simulink model "Model_3_Hieu_1_12"  (R2021a)
settings: Solver=VariableStepAuto  StartTime=0.0  StopTime=10  RelTol=1e-3
InitFcn:
  | ml=0.2;
  | mc=0.5;
  | mt=0.5;
  | g=9.81;
  | l_ref=0.5;
  | l_ini=0.5;
  | l=l_ini;
  | n1=5;n2=1;
  | x_ref=10;
  | 
  | %ADRC' s parameter caculation
  | %b0 = (ml+mc)/(mc*ml +mc*mt+ml*mt); %Hieu
  | b0=(ml+mc)/(mt*mc+2*ml*mc+mt*ml+ml^2+mc^2); %Enhanced-coupling
  | k_ESO = 50;
  | T_set  = 6;
  | 
  | s_cl = -5.85/T_set;
  | Kp   = s_cl^2;
  | Kd   = -2*s_cl;
  | 
  | s_ESO = k_ESO*s_cl;
  | l1        = -3*s_ESO;
  | l2        = 3*( s_ESO)^2;
  | l3        = -(s_ESO)^3;
  | 
  | %Observer
  | A = [-l1, 1, 0;
  |         -l2, 0, 1;
  |         -l3, 0, 0];
  | B = [0;
  |         b0;
  |         0];
  | L = [l1;
  |        l2;
  |        l3];
  | 
  | %b1 = (mt+mc)/(mc*ml +mc*mt+ml*mt);
  | b1=1/(ml+mc);
  | k_ESO1 =100;
  | T_set1  = 3;
  | s_cl1 = -5.85/T_set1;
  | Kp1   = s_cl1^2;
  | Kd1   = -2*s_cl1;
  | 
  | s_ESO1 = k_ESO1*s_cl1;
  | l11        = -3*s_ESO1;
  | l21        = 3*( s_ESO1)^2;
  | l31        = -(s_ESO1)^3;
  | 
  | %Observer
  | A1 = [-l11, 1, 0;
  |         -l21, 0, 1;
  |         -l31, 0, 0];
  | B1 = [0;
  |         b1;
  |         0];
  | L1 = [l11;
  |        l21;
  |        l31];
  | 
  | ... (+35 lines)
values from neighbouring files (symbols this model uses):
  particle = repmat(empty_particle, nPop, 1)    [PSO16_12.m]    (also in PSO_ZVD.m)
undefined symbols (not defined in the file or in its folder): i
libraries: neural x35, simulink_extras x11, simulink x5
(part 12 of 15)

== matlab function Model_3_Hieu_1_12/test_RBF_1 PSO/con lắc đôi2/Crane ==
  data: dx1 output; d1x input; l1 input; d1l1 input; the1 input; d1the1 input; the2 input; d1the2 input; Fx input; Fl input; dx2 output; dx3 output; dx4 output; dx5 output; dx6 output; m2 input; dx7 output; dx8 output
function [dx1,dx2,dx3,dx4,dx5,dx6,dx7,dx8] = fcn(d1x,l1,d1l1,the1,d1the1,the2,d1the2,Fx,Fl,m2)
 m =5; m1 =2; g =9.81; l2=0.5;

 dx1=d1x;

 dx2 = (Fx*m2*cos(the1 - the2)^2 - Fx*m2 - Fx*m1 + Fx*m2*sin(the1 - the2)^2 + Fl*m1*sin(the1) + Fl*m2*sin(the1) - Fl*m2*sin(the1 - the2)*cos(the2) - d1the2^2*l2*m2^2*sin(the2) - g*m2^2*cos(the2)*sin(the2) - Fl*m2*cos(the1 - the2)^2*sin(the1) - g*m2^2*cos(the1 - the2)*sin(the1 - the2)*sin(the1)^2 + Fl*m2*cos(the1 - the2)*sin(the1 - the2)*cos(the1) + d1the2^2*l2*m2^2*cos(the1 - the2)*sin(the1) - d1the2^2*l2*m2^2*sin(the1 - the2)*cos(the1) - d1the2^2*l2*m1*m2*sin(the2) + g*m2^2*cos(the1 - the2)*cos(the1)*sin(the2) + g*m2^2*cos(the1 - the2)*cos(the2)*sin(the1) - g*m2^2*sin(the1 - the2)*cos(the1)*cos(the2) - g*m1*m2*cos(the2)*sin(the2) + g*m2^2*sin(the1 - the2)*sin(the1)*sin(the2) + d1the2^2*l2*m2^2*cos(the1 - the2)^2*sin(the2) - d1the2^2*l2*m2^2*cos(the1 - the2)^3*sin(the1) + d1the2^2*l2*m2^2*sin(the1 - the2)^3*cos(the1) - g*m2^2*cos(the1 - the2)^2*cos(the1)*sin(the1) + d1the2^2*l2*m2^2*sin(the1 - the2)^2*sin(the2) + g*m2^2*sin(the1 - the2)^2*cos(the1)*sin(the1) + g*m2^2*cos(the1 - the2)*sin(the1 - the2)*cos(the1)^2 - g*m1*m2*cos(the1 - the2)*sin(the1 - the2)*sin(the1)^2 + d1the2^2*l2*m1*m2*cos(the1 - the2)*sin(the1) - d1the2^2*l2*m1*m2*sin(the1 - the2)*cos(the1) + g*m1*m2*cos(the1 - the2)*cos(the1)*sin(the2) + g*m1*m2*cos(the1 - the2)*cos(the2)*sin(the1) - g*m1*m2*sin(the1 - the2)*cos(the1)*cos(the2) + g*m1*m2*sin(the1 - the2)*sin(the1)*sin(the2) + d1the2^2*l2*m2^2*cos(the1 - the2)^2*sin(the1 - the2)*cos(the1) - d1the2^2*l2*m2^2*cos(the1 - the2)*sin(the1 - the2)^2*sin(the1) - g*m1*m2*cos(the1 - the2)^2*cos(the1)*sin(the1) + g*m1*m2*sin(the1 - the2)^2*cos(the1)*sin(the1) + g*m1*m2*cos(the1 - the2)*sin(the1 - the2)*cos(the1)^2)/(m1^2*cos(the1)^2 - m*m2 - 2*m1*m2 - m*m1 + m2^2*cos(the1)^2 + m2^2*cos(the2)^2 + m1^2*sin(the1)^2 + m2^2*sin(the1)^2 + m2^2*cos(the1 - the2)^2 + m2^2*sin(the1 - the2)^2 - m1^2 - m2^2 + 2*m1*m2*cos(the1)^2 + m1*m2*cos(the2)^2 + 2*m1*m2*sin(the1)^2 + m*m2*cos(the1 - the2)^2 + m1*m2*cos(the1 - the2)^2 + m*m2*sin(the1 - the2)^2 + m1*m2*sin(the1 - the2)^2 - m2^2*cos(the1 - the2)^2*sin(the1)^2 - m2^2*sin(the1 - the2)^2*cos(the1)^2 - 2*m2^2*sin(the1 - the2)*cos(the2)*sin(the1) - 2*m2^2*cos(the1 - the2)*cos(the1)*cos(the2) - m1*m2*cos(the1 - the2)^2*sin(the1)^2 - m1*m2*sin(the1 - the2)^2*cos(the1)^2 + 2*m2^2*cos(the1 - the2)*sin(the1 - the2)*cos(the1)*sin(the1) - 2*m1*m2*sin(the1 - the2)*cos(the2)*sin(the1) - 2*m1*m2*cos(the1 - the2)*cos(the1)*cos(the2) + 2*m1*m2*cos(the1 - the2)*sin(the1 - the2)*cos(the1)*sin(the1));

 %d2x = -(Fx*m1 + Fx*m2 + g*m1^2*sin(the1) + g*m2^2*sin(the1) - Fx*m2*cos(the1 - the2)^2 - Fx*m2*sin(the1 - the2)^2 - Fl*m1*sin(the1) - Fl*m2*sin(the1) + Fl*m2*sin(the1 - the2)*cos(the2) + d1the2^2*l2*m2^2*sin(the2) - g*m1^2*cos(the1)*sin(the1) - g*m2^2*cos(the1)*sin(the1) + g*m2^2*cos(the2)*sin(the2) + Fl*m2*cos(the1 - the2)^2*sin(the1) - g*m2^2*sin(the1 - the2)*cos(the2) + 2*g*m1*m2*sin(the1) - g*m2^2*cos(the1 - the2)^2*sin(the1) - Fl*m2*cos(the1 - the2)*sin(the1 - the2)*cos(the1) + 2*d1l1*d1the1*m2^2*cos(the1 - the2)^2*cos(the1) - 2*d1l1*d1the1*m2^3*cos(the1 - the2)^2*cos(the1) + d1the2^2*l2*m2^2*cos(the1 - the2)*sin(the1) + d1the2^2*l2*m2^2*sin(the1 - the2)*cos(the1) + d1the2^2*l2*m1*m2*sin(the2) - g*m2^2*cos(the1 - the2)*cos(the1)*sin(the2) + g*m2^2*sin(the1 - the2)*cos(the1)*cos(the2) - 2*g*m1*m2*cos(the1)*sin(the1) + g*m1*m2*cos(the2)*sin(the2) - g*m2^2*sin(the1 - the2)*sin(the1)*sin(the2) + g*m2^2*cos(the1 - the2)*sin(the1 - the2)*cos(the1) - g*m1*m2*sin(the1 - the2)*cos(the2) - d1the2^2*l2*m2^2*cos(the1 - the2)^2*sin(the2) - d1the2^2*l2*m2^2*cos(the1 - the2)^3*sin(the1) - d1the2^2*l2*m2^2*sin(the1 - the2)^3*cos(the1) + g*m2^2*cos(the1 - the2)^2*cos(the1)*sin(the1) - d1the2^2*l2*m2^2*sin(the1 - the2)^2*sin(the2) - 2*d1l1*d1the1*m2^2*cos(the1 - the2)*cos(the2) + 2*d1l1*d1the1*m2^3*cos(the1 - the2)*cos(the2) - g*m2^2*cos(the1 - the2)*sin(the1 - the2)*cos(the1)^2 - g*m1*m2*cos(the1 - the2)^2*sin(the1) + 2*d1l1*d1the1*m2^2*cos(the1 - the2)*sin(the1 - the2)*sin(the1) - 2*d1l1*d1the1*m2^3*cos(the1 - the2)*sin(the1 - the2)*sin(the1) + 2*d1l1*d1the1*m1*m2*cos(the1 - the2)^2*cos(the1) + 2*d1l1*d1the1*m1*m2^2*cos(the1 - the2)*cos(the2) - 2*d1the2^2*l2*m2^2*cos(the1 - the2)*sin(the1 - the2)*cos(the2) + d1the2^2*l2*m1*m2*cos(the1 - the2)*sin(the1) + d1the2^2*l2*m1*m2*sin(the1 - the2)*cos(the1) - g*m1*m2*cos(the1 - the2)*cos(the1)*sin(the2) + g*m1*m2*sin(the1 - the2)*cos(the1)*cos(the2) - g*m1*m2*sin(the1 - the2)*sin(the1)*sin(the2) + g*m1*m2*cos(the1 - the2)*sin(the1 - the2)*cos(the1) - 2*d1l1*d1the1*m1*m2^2*cos(the1 - the2)^2*cos(the1) + d1the2^2*l2*m2^2*cos(the1 - the2)^2*sin(the1 - the2)*cos(the1) + d1the2^2*l2*m2^2*cos(the1 - the2)*sin(the1 - the2)^2*sin(the1) + g*m1*m2*cos(the1 - the2)^2*cos(the1)*sin(the1) - 2*d1l1*d1the1*m1*m2*cos(the1 - the2)*cos(the2) - g*m1*m2*cos(the1 - the2)*sin(the1 - the2)*cos(the1)^2 + 2*d1l1*d1the1*m1*m2*cos(the1 - the2)*sin(the1 - the2)*sin(the1) - 2*d1l1*d1the1*m1*m2^2*cos(the1 - the2)*sin(the1 - the2)*sin(the1))/(m1^2*cos(the1)^2 - m*m2 - 2*m1*m2 - m*m1 + m2^2*cos(the1)^2 + m2^2*cos(the2)^2 + m1^2*sin(the1)^2 + m2^2*sin(the1)^2 + m2^2*cos(the1 - the2)^2 + m2^2*sin(the1 - the2)^2 - m1^2 - m2^2 + 2*m1*m2*cos(the1)^2 + m1*m2*cos(the2)^2 + 2*m1*m2*sin(the1)^2 + m*m2*cos(the1 - the2)^2 + m1*m2*cos(the1 - the2)^2 + m*m2*sin(the1 - the2)^2 + m1*m2*sin(the1 - the2)^2 - m2^2*cos(the1 - the2)^2*sin(the1)^2 - m2^2*sin(the1 - the2)^2*cos(the1)^2 - 2*m2^2*sin(the1 - the2)*cos(the2)*sin(the1) - 2*m2^2*cos(the1 - the2)*cos(the1)*cos(the2) - m1*m2*cos(the1 - the2)^2*sin(the1)^2 - m1*m2*sin(the1 - the2)^2*cos(the1)^2 + 2*m2^2*cos(the1 - the2)*sin(the1 - the2)*cos(the1)*sin(the1) - 2*m1*m2*sin(the1 - the2)*cos(the2)*sin(the1) - 2*m1*m2*cos(the1 - the2)*cos(the1)*cos(the2) + 2*m1*m2*cos(the1 - the2)*sin(the1 - the2)*cos(the1)*sin(the1));

 dx3=d1l1;

 dx4 = (Fx*m1^2*sin(the1) - Fl*m2^2 - Fl*m1^2 + Fx*m2^2*sin(the1) - d1the1^2*l1*m1^3 - d1the1^2*l1*m2^3 - g*m1^3*cos(the1) - g*m2^3*cos(the1) - Fl*m*m1 - Fl*m*m2 - 2*Fl*m1*m2 + Fl*m1^2*cos(the1)^2 + Fl*m2^2*cos(the1)^2 + Fl*m2^2*cos(the2)^2 + g*m1^3*cos(the1)^3 + g*m2^3*cos(the1)^3 + Fl*m2^2*cos(the1 - the2)^2 + 3*g*m1*m2^2*cos(the1)^3 + 3*g*m1^2*m2*cos(the1)^3 - Fx*m2^2*sin(the1 - the2)*cos(the2) - d1the2^2*l2*m2^3*cos(the1 - the2) + 2*Fx*m1*m2*sin(the1) + d1the1^2*l1*m1^3*cos(the1)^2 + d1the1^2*l1*m2^3*cos(the1)^2 + d1the1^2*l1*m2^3*cos(the2)^2 - g*m2^3*sin(the1 - the2)*sin(the2) + g*m2^3*cos(the1)*cos(the2)^2 + d1the1^2*l1*m1^3*sin(the1)^2 + d1the1^2*l1*m2^3*sin(the1)^2 + g*m1^3*cos(the1)*sin(the1)^2 + g*m2^3*cos(the1)*sin(the1)^2 + 2*Fl*m1*m2*cos(the1)^2 + Fl*m1*m2*cos(the2)^2 - Fx*m2^2*cos(the1 - the2)^2*sin(the1) + d1the1^2*l1*m2^3*cos(the1 - the2)^2 + d1the2^2*l2*m2^3*cos(the1 - the2)^3 - d1the1^2*l1*m*m1^2 - d1the1^2*l1*m*m2^2 - 3*d1the1^2*l1*m1*m2^2 - 3*d1the1^2*l1*m1^2*m2 + g*m2^3*cos(the1 - the2)^2*cos(the1) + d1the1^2*l1*m2^3*sin(the1 - the2)^2 - g*m*m1^2*cos(the1) - g*m*m2^2*cos(the1) - 3*g*m1*m2^2*cos(the1) - 3*g*m1^2*m2*cos(the1) + Fl*m*m2*cos(the1 - the2)^2 + Fl*m1*m2*cos(the1 - the2)^2 - g*m*m2^2*sin(the1 - the2)*sin(the2) - 2*g*m1*m2^2*sin(the1 - the2)*sin(the2) - g*m1^2*m2*sin(the1 - the2)*sin(the2) - d1the1^2*l1*m2^3*cos(the1 - the2)^2*sin(the1)^2 - d1the1^2*l1*m2^3*sin(the1 - the2)^2*cos(the1)^2 + 2*g*m1*m2^2*cos(the1)*cos(the2)^2 + g*m1^2*m2*cos(the1)*cos(the2)^2 + 3*d1the1^2*l1*m1*m2^2*sin(the1)^2 + 3*d1the1^2*l1*m1^2*m2*sin(the1)^2 + 3*g*m1*m2^2*cos(the1)*sin(the1)^2 + 3*g*m1^2*m2*cos(the1)*sin(the1)^2 + d1the2^2*l2*m2^3*sin(the1)*sin(the2) - 2*Fl*m2^2*cos(the1 - the2)*cos(the1)*cos(the2) + d1the1^2*l1*m*m2^2*cos(the1 - the2)^2 + 2*d1the1^2*l1*m1*m2^2*cos(the1 - the2)^2 + d1the1^2*l1*m1^2*m2*cos(the1 - the2)^2 + d1the2^2*l2*m*m2^2*cos(the1 - the2)^3 + d1the2^2*l2*m1*m2^2*cos(the1 - the2)^3 + g*m2^3*cos(the2)*sin(the1)*sin(the2) + g*m*m2^2*cos(the1 - the2)^2*cos(the1) + 2*g*m1*m2^2*cos(the1 - the2)^2*cos(the1) + g*m1^2*m2*cos(the1 - the2)^2*cos(the1) + d1the1^2*l1*m*m2^2*sin(the1 - the2)^2 + 2*d1the1^2*l1*m1*m2^2*sin(the1 - the2)^2 + d1the1^2*l1*m1^2*m2*sin(the1 - the2)^2 + Fx*m2^2*cos(the1 - the2)*sin(the1 - the2)*cos(the1) - Fx*m1*m2*sin(the1 - the2)*cos(the2) + d1the2^2*l2*m2^3*cos(the1 - the2)*cos(the1)^2 + d1the2^2*l2*m2^3*cos(the1 - the2)*cos(the2)^2 + g*m2^3*cos(the1 - the2)*sin(the1 - the2)*sin(the1) - 2*g*m2^3*cos(the1 - the2)*cos(the1)^2*cos(the2) - g*m2^3*cos(the1 - the2)*cos(the2)*sin(the1)^2 + g*m2^3*sin(the1 - the2)*cos(the1)^2*sin(the2) - Fx*m1*m2*cos(the1 - the2)^2*sin(the1) - d1the2^2*l2*m*m2^2*cos(the1 - the2) - 2*d1the2^2*l2*m1*m2^2*cos(the1 - the2) - d1the2^2*l2*m1^2*m2*cos(the1 - the2) - 2*d1the1^2*l1*m*m1*m2 + d1the2^2*l2*m2^3*cos(the1 - the2)*sin(the1 - the2)^2 - 2*g*m*m1*m2*cos(the1) + 3*d1the1^2*l1*m1*m2^2*cos(the1)^2 + 3*d1the1^2*l1*m1^2*m2*cos(the1)^2 + 2*d1the1^2*l1*m1*m2^2*cos(the2)^2 + d1the1^2*l1*m1^2*m2*cos(the2)^2 + 2*d1the2^2*l2*m1*m2^2*cos(the1 - the2)*cos(the1)^2 + d1the2^2*l2*m1^2*m2*cos(the1 - the2)*cos(the1)^2 + d1the2^2*l2*m1*m2^2*cos(the1 - the2)*cos(the2)^2 + g*m*m2^2*cos(the1 - the2)*sin(the1 - the2)*sin(the1) + 2*g*m1*m2^2*cos(the1 - the2)*sin(the1 - the2)*sin(the1) + g*m1^2*m2*cos(the1 - the2)*sin(the1 - the2)*sin(the1) - g*m*m1*m2*sin(the1 - the2)*sin(the2) - 2*d1the1^2*l1*m2^3*cos(the1 - the2)*cos(the1)*cos(the2) - 4*g*m1*m2^2*cos(the1 - the2)*cos(the1)^2*cos(the2) - 2*g*m1^2*m2*cos(the1 - the2)*cos(the1)^2*cos(the2) - 2*g*m1*m2^2*cos(the1 - the2)*cos(the2)*sin(the1)^2 - g*m1^2*m2*cos(the1 - the2)*cos(the2)*sin(the1)^2 - 2*d1the1^2*l1*m2^3*sin(the1 - the2)*cos(the2)*sin(the1) + d1the2^2*l2*m2^3*sin(the1 - the2)*cos(the1)*sin(the1) - d1the2^2*l2*m2^3*sin(the1 - the2)*cos(the2)*sin(the2) + 2*g*m1*m2^2*sin(the1 - the2)*cos(the1)^2*sin(the2) + g*m1^2*m2*sin(the1 - the2)*cos(the1)^2*sin(the2) - 2*Fl*m1*m2*cos(the1 - the2)*cos(the1)*cos(the2) + d1the1^2*l1*m*m1*m2*cos(the1 - the2)^2 - g*m2^3*cos(the1 - the2)*cos(the1)*sin(the1)*sin(the2) - g*m2^3*sin(the1 - the2)*cos(the1)*cos(the2)*sin(the1) + d1the2^2*l2*m*m2^2*cos(the1 - the2)*sin(the1 - the2)^2 + d1the2^2*l2*m1*m2^2*cos(the1 - the2)*sin(the1 - the2)^2 + g*m*m1*m2*cos(the1 - the2)^2*cos(the1) + d1the1^2*l1*m*m1*m2*sin(the1 - the2)^2 - 2*d1the2^2*l2*m2^3*cos(the1 - the2)^2*cos(the1)*cos(the2) - 2*d1the1^2*l1*m1*m2^2*cos(the1 - the2)^2*sin(the1)^2 - 2*d1the1^2*l1*m1*m2^2*sin(the1 - the2)^2*cos(the1)^2 - d1the1^2*l1*m1^2*m2*cos(the1 - the2)^2*sin(the1)^2 - d1the1^2*l1*m1^2*m2*sin(the1 - the2)^2*cos(the1)^2 + Fx*m1*m2*cos(the1 - the2)*sin(the1 - the2)*cos(the1) - d1the2^2*l2*m2^3*sin(the1 - the2)^2*cos(the1)*cos(the2) - d1the2^2*l2*m2^3*cos(the1 - the2)^2*sin(the1)*sin(the2) + 2*d1the2^2*l2*m1*m2^2*sin(the1)*sin(the2) + d1the2^2*l2*m1^2*m2*sin(the1)*sin(the2) + 2*g*m1*m2^2*cos(the2)*sin(the1)*sin(the2) + g*m1^2*m2*cos(the2)*sin(the1)*sin(the2) - d1the2^2*l2*m*m1*m2*cos(the1 - the2) - d1the2^2*l2*m1*m2^2*cos(the1 - the2)^2*sin(the1)*sin(the2) + g*m*m1*m2*cos(the1 - the2)*sin(the1 - the2)*sin(the1) + 2*d1the1^2*l1*m2^3*cos(the1 - the2)*sin(the1 - the2)*cos(the1)*sin(the1) + d1the2^2*l2*m2^3*cos(the1 - the2)*sin(the1 - the2)*cos(the1)*sin(the2) - d1the2^2*l2*m2^3*cos(the1 - the2)*sin(the1 - the2)*cos(the2)*sin(the1) - 4*d1the1^2*l1*m1*m2^2*cos(the1 - the2)*cos(the1)*cos(the2) - 2*d1the1^2*l1*m1^2*m2*cos(the1 - the2)*cos(the1)*cos(the2) - 4*d1the1^2*l1*m1*m2^2*sin(the1 - the2)*cos(the2)*sin(the1) - 2*d1the1^2*l1*m1^2*m2*sin(the1 - the2)*cos(the2)*sin(the1) + 2*d1the2^2*l2*m1*m2^2*sin(the1 - the2)*cos(the1)*sin(the1) + d1the2^2*l2*m1^2*m2*sin(the1 - the2)*cos(the1)*sin(the1) - d1the2^2*l2*m1*m2^2*sin(the1 - the2)*cos(the2)*sin(the2) - 2*g*m1*m2^2*cos(the1 - the2)*cos(the1)*sin(the1)*sin(the2) - 2*g*m1*m2^2*sin(the1 - the2)*cos(the1)*cos(the2)*sin(the1) - g*m1^2*m2*cos(the1 - the2)*cos(the1)*sin(the1)*sin(the2) - g*m1^2*m2*sin(the1 - the2)*cos(the1)*cos(the2)*sin(the1) - 2*d1the2^2*l2*m1*m2^2*cos(the1 - the2)^2*cos(the1)*cos(the2) - d1the2^2*l2*m1*m2^2*sin(the1 - the2)^2*cos(the1)*cos(the2) + 4*d1the1^2*l1*m1*m2^2*cos(the1 - the2)*sin(the1 - the2)*cos(the1)*sin(the1) + 2*d1the1^2*l1*m1^2*m2*cos(the1 - the2)*sin(the1 - the2)*cos(the1)*sin(the1) + d1the2^2*l2*m1*m2^2*cos(the1 - the2)*sin(the1 - the2)*cos(the1)*sin(the2) - d1the2^2*l2*m1*m2^2*cos(the1 - the2)*sin(the1 - the2)*cos(the2)*sin(the1))/((m1 + m2)*(m1^2*cos(the1)^2 - m*m2 - 2*m1*m2 - m*m1 + m2^2*cos(the1)^2 + m2^2*cos(the2)^2 + m1^2*sin(the1)^2 + m2^2*sin(the1)^2 + m2^2*cos(the1 - the2)^2 + m2^2*sin(the1 - the2)^2 - m1^2 - m2^2 + 2*m1*m2*cos(the1)^2 + m1*m2*cos(the2)^2 + 2*m1*m2*sin(the1)^2 + m*m2*cos(the1 - the2)^2 + m1*m2*cos(the1 - the2)^2 + m*m2*sin(the1 - the2)^2 + m1*m2*sin(the1 - the2)^2 - m2^2*cos(the1 - the2)^2*sin(the1)^2 - m2^2*sin(the1 - the2)^2*cos(the1)^2 - 2*m2^2*sin(the1 - the2)*cos(the2)*sin(the1) - 2*m2^2*cos(the1 - the2)*cos(the1)*cos(the2) - m1*m2*cos(the1 - the2)^2*sin(the1)^2 - m1*m2*sin(the1 - the2)^2*cos(the1)^2 + 2*m2^2*cos(the1 - the2)*sin(the1 - the2)*cos(the1)*sin(the1) - 2*m1*m2*sin(the1 - the2)*cos(the2)*sin(the1) - 2*m1*m2*cos(the1 - the2)*cos(the1)*cos(the2) + 2*m1*m2*cos(the1 - the2)*sin(the1 - the2)*cos(the1)*sin(the1)));

 %dx4 = (g*m1^3 - Fl*m2^2 - Fl*m1^2 + g*m2^3 + Fx*m1^2*sin(the1) + Fx*m2^2*sin(the1) - d1the1^2*l1*m1^3 - d1the1^2*l1*m2^3 - g*m1^3*cos(the1) - g*m2^3*cos(the1) - Fl*m*m1 - Fl*m*m2 - 2*Fl*m1*m2 + Fl*m1^2*cos(the1)^2 + Fl*m2^2*cos(the1)^2 + Fl*m2^2*cos(the2)^2 - g*m1^3*cos(the1)^2 + g*m1^3*cos(the1)^3 - g*m2^3*cos(the1)^2 + g*m2^3*cos(the1)^3 - g*m2^3*cos(the2)^2 + Fl*m2^2*cos(the1 - the2)^2 - g*m2^3*cos(the1 - the2)^2 + g*m*m1^2 + g*m*m2^2 + 3*g*m1*m2^2 + 3*g*m1^2*m2 + 2*g*m*m1*m2 - 3*g*m1*m2^2*cos(the1)^2 - 3*g*m1^2*m2*cos(the1)^2 + 3*g*m1*m2^2*cos(the1)^3 - 2*g*m1*m2^2*cos(the2)^2 + 3*g*m1^2*m2*cos(the1)^3 - g*m1^2*m2*cos(the2)^2 - Fx*m2^2*sin(the1 - the2)*cos(the2) + d1the2^2*l2*m2^3*cos(the1 - the2) + 2*Fx*m1*m2*sin(the1) - g*m*m2^2*cos(the1 - the2)^2 - 2*g*m1*m2^2*cos(the1 - the2)^2 - g*m1^2*m2*cos(the1 - the2)^2 + d1the1^2*l1*m1^3*cos(the1)^2 + d1the1^2*l1*m2^3*cos(the1)^2 + d1the1^2*l1*m2^3*cos(the2)^2 - g*m2^3*sin(the1 - the2)*sin(the2) + g*m2^3*cos(the1)*cos(the2)^2 + d1the1^2*l1*m1^3*sin(the1)^2 + d1the1^2*l1*m2^3*sin(the1)^2 + 2*Fl*m1*m2*cos(the1)^2 + Fl*m1*m2*cos(the2)^2 - Fx*m2^2*cos(the1 - the2)^2*sin(the1) + d1the1^2*l1*m2^3*cos(the1 - the2)^2 - d1the2^2*l2*m2^3*cos(the1 - the2)^3 - d1the1^2*l1*m*m1^2 - d1the1^2*l1*m*m2^2 - 3*d1the1^2*l1*m1*m2^2 - 3*d1the1^2*l1*m1^2*m2 + g*m2^3*cos(the1 - the2)^2*cos(the1) + d1the1^2*l1*m2^3*sin(the1 - the2)^2 - g*m*m1^2*cos(the1) - g*m*m2^2*cos(the1) - 3*g*m1*m2^2*cos(the1) - 3*g*m1^2*m2*cos(the1) + Fl*m*m2*cos(the1 - the2)^2 + Fl*m1*m2*cos(the1 - the2)^2 - g*m*m2^2*sin(the1 - the2)*sin(the2) - 2*g*m1*m2^2*sin(the1 - the2)*sin(the2) - g*m1^2*m2*sin(the1 - the2)*sin(the2) - d1the1^2*l1*m2^3*cos(the1 - the2)^2*sin(the1)^2 - d1the1^2*l1*m2^3*sin(the1 - the2)^2*cos(the1)^2 + 2*g*m1*m2^2*cos(the1)*cos(the2)^2 + g*m1^2*m2*cos(the1)*cos(the2)^2 + 3*d1the1^2*l1*m1*m2^2*sin(the1)^2 + 3*d1the1^2*l1*m1^2*m2*sin(the1)^2 + 2*d1l1*d1the1*m2^3*cos(the1 - the2)*sin(the1 - the2) - 2*d1l1*d1the1*m2^4*cos(the1 - the2)*sin(the1 - the2) + d1the2^2*l2*m2^3*sin(the1)*sin(the2) - 2*Fl*m2^2*cos(the1 - the2)*cos(the1)*cos(the2) + d1the1^2*l1*m*m2^2*cos(the1 - the2)^2 + 2*d1the1^2*l1*m1*m2^2*cos(the1 - the2)^2 + d1the1^2*l1*m1^2*m2*cos(the1 - the2)^2 - d1the2^2*l2*m*m2^2*cos(the1 - the2)^3 - d1the2^2*l2*m1*m2^2*cos(the1 - the2)^3 + g*m2^3*cos(the2)*sin(the1)*sin(the2) + g*m*m2^2*cos(the1 - the2)^2*cos(the1) + 2*g*m1*m2^2*cos(the1 - the2)^2*cos(the1) + g*m1^2*m2*cos(the1 - the2)^2*cos(the1) + d1the1^2*l1*m*m2^2*sin(the1 - the2)^2 + 2*d1the1^2*l1*m1*m2^2*sin(the1 - the2)^2 + d1the1^2*l1*m1^2*m2*sin(the1 - the2)^2 + 2*g*m2^3*cos(the1 - the2)*cos(the1)*cos(the2) + Fx*m2^2*cos(the1 - the2)*sin(the1 - the2)*cos(the1) - Fx*m1*m2*sin(the1 - the2)*cos(the2) - g*m*m1*m2*cos(the1 - the2)^2 - d1the2^2*l2*m2^3*cos(the1 - the2)*cos(the1)^2 - d1the2^2*l2*m2^3*cos(the1 - the2)*cos(the2)^2 - 2*g*m2^3*cos(the1 - the2)*cos(the1)^2*cos(the2) + g*m2^3*sin(the1 - the2)*cos(the1)^2*sin(the2) - Fx*m1*m2*cos(the1 - the2)^2*sin(the1) + d1the2^2*l2*m*m2^2*cos(the1 - the2) + 2*d1the2^2*l2*m1*m2^2*cos(the1 - the2) + d1the2^2*l2*m1^2*m2*cos(the1 - the2) - 2*d1the1^2*l1*m*m1*m2 + d1the2^2*l2*m2^3*cos(the1 - the2)*sin(the1 - the2)^2 - 2*g*m*m1*m2*cos(the1) + 3*d1the1^2*l1*m1*m2^2*cos(the1)^2 + 3*d1the1^2*l1*m1^2*m2*cos(the1)^2 + 2*d1the1^2*l1*m1*m2^2*cos(the2)^2 + d1the1^2*l1*m1^2*m2*cos(the2)^2 - 2*d1the2^2*l2*m1*m2^2*cos(the1 - the2)*cos(the1)^2 - d1the2^2*l2*m1^2*m2*cos(the1 - the2)*cos(the1)^2 - d1the2^2*l2*m1*m2^2*cos(the1 - the2)*cos(the2)^2 - g*m*m1*m2*sin(the1 - the2)*sin(the2) - 2*d1the1^2*l1*m2^3*cos(the1 - the2)*cos(the1)*cos(the2) - 4*g*m1*m2^2*cos(the1 - the2)*cos(the1)^2*cos(the2) - 2*g*m1^2*m2*cos(the1 - the2)*cos(the1)^2*cos(the2) + 2*d1l1*d1the1*m2^3*cos(the1 - the2)^2*cos(the1)*sin(the1) - 2*d1l1*d1the1*m2^4*cos(the1 - the2)^2*cos(the1)*sin(the1) - 2*d1the1^2*l1*m2^3*sin(the1 - the2)*cos(the2)*sin(the1) + d1the2^2*l2*m2^3*sin(the1 - the2)*cos(the1)*sin(the1) - d1the2^2*l2*m2^3*sin(the1 - the2)*cos(the2)*sin(the2) + 2*g*m1*m2^2*sin(the1 - the2)*cos(the1)^2*sin(the2) + g*m1^2*m2*sin(the1 - the2)*cos(the1)^2*sin(the2) - 2*Fl*m1*m2*cos(the1 - the2)*cos(the1)*cos(the2) + d1the1^2*l1*m*m1*m2*cos(the1 - the2)^2 - g*m2^3*cos(the1 - the2)*cos(the1)*sin(the1)*sin(the2) + d1the2^2*l2*m*m2^2*cos(the1 - the2)*sin(the1 - the2)^2 + d1the2^2*l2*m1*m2^2*cos(the1 - the2)*sin(the1 - the2)^2 + g*m*m1*m2*cos(the1 - the2)^2*cos(the1) + d1the1^2*l1*m*m1*m2*sin(the1 - the2)^2 - 2*d1l1*d1the1*m2^3*cos(the1 - the2)*sin(the1 - the2)*cos(the1)^2 + 2*d1l1*d1the1*m2^4*cos(the1 - the2)*sin(the1 - the2)*cos(the1)^2 + 2*d1the2^2*l2*m2^3*cos(the1 - the2)^2*cos(the1)*cos(the2) - 2*d1the1^2*l1*m1*m2^2*cos(the1 - the2)^2*sin(the1)^2 - 2*d1the1^2*l1*m1*m2^2*sin(the1 - the2)^2*cos(the1)^2 - d1the1^2*l1*m1^2*m2*cos(the1 - the2)^2*sin(the1)^2 - d1the1^2*l1*m1^2*m2*sin(the1 - the2)^2*cos(the1)^2 + Fx*m1*m2*cos(the1 - the2)*sin(the1 - the2)*cos(the1) - d1the2^2*l2*m2^3*sin(the1 - the2)^2*cos(the1)*cos(the2) + 2*d1l1*d1the1*m*m2^2*cos(the1 - the2)*sin(the1 - the2) - 2*d1l1*d1the1*m*m2^3*cos(the1 - the2)*sin(the1 - the2) + 4*d1l1*d1the1*m1*m2^2*cos(the1 - the2)*sin(the1 - the2) + 2*d1l1*d1the1*m1^2*m2*cos(the1 - the2)*sin(the1 - the2) - 4*d1l1*d1the1*m1*m2^3*cos(the1 - the2)*sin(the1 - the2) - d1the2^2*l2*m2^3*cos(the1 - the2)^2*sin(the1)*sin(the2) + 2*d1the2^2*l2*m1*m2^2*sin(the1)*sin(the2) + d1the2^2*l2*m1^2*m2*sin(the1)*sin(the2) + 2*g*m1*m2^2*cos(the2)*sin(the1)*sin(the2) + g*m1^2*m2*cos(the2)*sin(the1)*sin(the2) + 4*g*m1*m2^2*cos(the1 - the2)*cos(the1)*cos(the2) + 2*g*m1^2*m2*cos(the1 - the2)*cos(the1)*cos(the2) - 2*d1l1*d1the1*m2^3*cos(the1 - the2)*cos(the2)*sin(the1) + 2*d1l1*d1the1*m2^4*cos(the1 - the2)*cos(the2)*sin(the1) + d1the2^2*l2*m*m1*m2*cos(the1 - the2) - 2*d1l1*d1the1*m1^2*m2^2*cos(the1 - the2)*sin(the1 - the2) - d1the2^2*l2*m1*m2^2*cos(the1 - the2)^2*sin(the1)*sin(the2) + 2*d1l1*d1the1*m1^2*m2^2*cos(the1 - the2)*sin(the1 - the2)*cos(the1)^2 - 4*d1l1*d1the1*m1*m2^2*cos(the1 - the2)*cos(the2)*sin(the1) - 2*d1l1*d1the1*m1^2*m2*cos(the1 - the2)*cos(the2)*sin(the1) + 4*d1l1*d1the1*m1*m2^3*cos(the1 - the2)*cos(the2)*sin(the1) + 2*d1the1^2*l1*m2^3*cos(the1 - the2)*sin(the1 - the2)*cos(the1)*sin(the1) + d1the2^2*l2*m2^3*cos(the1 - the2)*sin(the1 - the2)*cos(the1)*sin(the2) - d1the2^2*l2*m2^3*cos(the1 - the2)*sin(the1 - the2)*cos(the2)*sin(the1) - 4*d1the1^2*l1*m1*m2^2*cos(the1 - the2)*cos(the1)*cos(the2) - 2*d1the1^2*l1*m1^2*m2*cos(the1 - the2)*cos(the1)*cos(the2) + 4*d1l1*d1the1*m1*m2^2*cos(the1 - the2)^2*cos(the1)*sin(the1) + 2*d1l1*d1the1*m1^2*m2*cos(the1 - the2)^2*cos(the1)*sin(the1) - 4*d1l1*d1the1*m1*m2^3*cos(the1 - the2)^2*cos(the1)*sin(the1) + 2*d1l1*d1the1*m1^2*m2^2*cos(the1 - the2)*cos(the2)*sin(the1) + 2*d1l1*d1the1*m*m1*m2*cos(the1 - the2)*sin(the1 - the2) - 4*d1the1^2*l1*m1*m2^2*sin(the1 - the2)*cos(the2)*sin(the1) - 2*d1the1^2*l1*m1^2*m2*sin(the1 - the2)*cos(the2)*sin(the1) + 2*d1the2^2*l2*m1*m2^2*sin(the1 - the2)*cos(the1)*sin(the1) + d1the2^2*l2*m1^2*m2*sin(the1 - the2)*cos(the1)*sin(the1) - d1the2^2*l2*m1*m2^2*sin(the1 - the2)*cos(the2)*sin(the2) - 2*g*m1*m2^2*cos(the1 - the2)*cos(the1)*sin(the1)*sin(the2) - g*m1^2*m2*cos(the1 - the2)*cos(the1)*sin(the1)*sin(the2) - 4*d1l1*d1the1*m1*m2^2*cos(the1 - the2)*sin(the1 - the2)*cos(the1)^2 - 2*d1l1*d1the1*m1^2*m2*cos(the1 - the2)*sin(the1 - the2)*cos(the1)^2 + 4*d1l1*d1the1*m1*m2^3*cos(the1 - the2)*sin(the1 - the2)*cos(the1)^2 + 2*d1the2^2*l2*m1*m2^2*cos(the1 - the2)^2*cos(the1)*cos(the2) - 2*d1l1*d1the1*m1^2*m2^2*cos(the1 - the2)^2*cos(the1)*sin(the1) - d1the2^2*l2*m1*m2^2*sin(the1 - the2)^2*cos(the1)*cos(the2) - 2*d1l1*d1the1*m*m1*m2^2*cos(the1 - the2)*sin(the1 - the2) + 4*d1the1^2*l1*m1*m2^2*cos(the1 - the2)*sin(the1 - the2)*cos(the1)*sin(the1) + 2*d1the1^2*l1*m1^2*m2*cos(the1 - the2)*sin(the1 - the2)*cos(the1)*sin(the1) + d1the2^2*l2*m1*m2^2*cos(the1 - the2)*sin(the1 - the2)*cos(the1)*sin(the2) - d1the2^2*l2*m1*m2^2*cos(the1 - the2)*sin(the1 - the2)*cos(the2)*sin(the1))/((m1 + m2)*(m1^2*cos(the1)^2 - m*m2 - 2*m1*m2 - m*m1 + m2^2*cos(the1)^2 + m2^2*cos(the2)^2 + m1^2*sin(the1)^2 + m2^2*sin(the1)^2 + m2^2*cos(the1 - the2)^2 + m2^2*sin(the1 - the2)^2 - m1^2 - m2^2 + 2*m1*m2*cos(the1)^2 + m1*m2*cos(the2)^2 + 2*m1*m2*sin(the1)^2 + m*m2*cos(the1 - the2)^2 + m1*m2*cos(the1 - the2)^2 + m*m2*sin(the1 - the2)^2 + m1*m2*sin(the1 - the2)^2 - m2^2*cos(the1 - the2)^2*sin(the1)^2 - m2^2*sin(the1 - the2)^2*cos(the1)^2 - 2*m2^2*sin(the1 - the2)*cos(the2)*sin(the1) - 2*m2^2*cos(the1 - the2)*cos(the1)*cos(the2) - m1*m2*cos(the1 - the2)^2*sin(the1)^2 - m1*m2*sin(the1 - the2)^2*cos(the1)^2 + 2*m2^2*cos(the1 - the2)*sin(the1 - the2)*cos(the1)*sin(the1) - 2*m1*m2*sin(the1 - the2)*cos(the2)*sin(the1) - 2*m1*m2*cos(the1 - the2)*cos(the1)*cos(the2) + 2*m1*m2*cos(the1 - the2)*sin(the1 - the2)*cos(the1)*sin(the1)));

 dx5=d1the1;
 
 dx6 = -(g*m1^3*sin(the1)^3 - Fx*m2^2*cos(the1) - g*m1^3*sin(the1) - g*m2^3*sin(the1) - Fx*m1^2*cos(the1) + g*m2^3*sin(the1)^3 - 2*d1l1*d1the1*m1^3 - 2*d1l1*d1the1*m2^3 + 2*d1l1*d1the1*m1^3*cos(the1)^2 + 2*d1l1*d1the1*m2^3*cos(the1)^2 + 2*d1l1*d1the1*m2^3*cos(the2)^2 + Fl*m1^2*cos(the1)*sin(the1) + Fl*m2^2*cos(the1)*sin(the1) + 2*d1l1*d1the1*m1^3*sin(the1)^2 + 2*d1l1*d1the1*m2^3*sin(the1)^2 + 3*g*m1*m2^2*sin(the1)^3 + 3*g*m1^2*m2*sin(the1)^3 + Fx*m2^2*cos(the1 - the2)*cos(the2) - 2*Fx*m1*m2*cos(the1) + 2*d1l1*d1the1*m2^3*cos(the1 - the2)^2 - 2*d1l1*d1the1*m*m1^2 - 2*d1l1*d1the1*m*m2^2 - 6*d1l1*d1the1*m1*m2^2 - 6*d1l1*d1the1*m1^2*m2 + 2*d1l1*d1the1*m2^3*sin(the1 - the2)^2 - d1the2^2*l2*m2^3*sin(the1 - the2) + g*m2^3*cos(the1 - the2)*sin(the2) + Fl*m2^2*cos(the1 - the2)*sin(the1 - the2) + g*m1^3*cos(the1)^2*sin(the1) + g*m2^3*cos(the1)^2*sin(the1) + g*m2^3*cos(the2)^2*sin(the1) + Fx*m2^2*sin(the1 - the2)^2*cos(the1) + d1the2^2*l2*m2^3*sin(the1 - the2)^3 - g*m*m1^2*sin(the1) - g*m*m2^2*sin(the1) - 3*g*m1*m2^2*sin(the1) - 3*g*m1^2*m2*sin(the1) + g*m2^3*sin(the1 - the2)^2*sin(the1) - d1the2^2*l2*m2^3*cos(the1)*sin(the2) + 3*g*m1*m2^2*cos(the1)^2*sin(the1) + 3*g*m1^2*m2*cos(the1)^2*sin(the1) + 2*g*m1*m2^2*cos(the2)^2*sin(the1) + g*m1^2*m2*cos(the2)^2*sin(the1) - g*m2^3*cos(the1)*cos(the2)*sin(the2) - Fl*m2^2*cos(the1 - the2)*cos(the2)*sin(the1) - Fl*m2^2*sin(the1 - the2)*cos(the1)*cos(the2) + 2*Fl*m1*m2*cos(the1)*sin(the1) + d1the2^2*l2*m*m2^2*sin(the1 - the2)^3 + d1the2^2*l2*m1*m2^2*sin(the1 - the2)^3 + g*m*m2^2*sin(the1 - the2)^2*sin(the1) + 2*g*m1*m2^2*sin(the1 - the2)^2*sin(the1) + g*m1^2*m2*sin(the1 - the2)^2*sin(the1) + Fx*m1*m2*cos(the1 - the2)*cos(the2) - 4*d1l1*d1the1*m*m1*m2 - Fx*m2^2*cos(the1 - the2)*sin(the1 - the2)*sin(the1) + g*m2^3*cos(the1 - the2)*sin(the1 - the2)*cos(the1) + 6*d1l1*d1the1*m1*m2^2*cos(the1)^2 + 6*d1l1*d1the1*m1^2*m2*cos(the1)^2 + 4*d1l1*d1the1*m1*m2^2*cos(the2)^2 + 2*d1l1*d1the1*m1^2*m2*cos(the2)^2 - 2*d1l1*d1the1*m2^3*cos(the1 - the2)^2*sin(the1)^2 - 2*d1l1*d1the1*m2^3*sin(the1 - the2)^2*cos(the1)^2 + Fl*m*m2*cos(the1 - the2)*sin(the1 - the2) + Fl*m1*m2*cos(the1 - the2)*sin(the1 - the2) + 6*d1l1*d1the1*m1*m2^2*sin(the1)^2 + 6*d1l1*d1the1*m1^2*m2*sin(the1)^2 + d1the2^2*l2*m2^3*sin(the1 - the2)*cos(the2)^2 - g*m2^3*sin(the1 - the2)*cos(the1)^2*cos(the2) + d1the2^2*l2*m2^3*sin(the1 - the2)*sin(the1)^2 + 2*d1l1*d1the1*m*m2^2*cos(the1 - the2)^2 + 4*d1l1*d1the1*m1*m2^2*cos(the1 - the2)^2 + 2*d1l1*d1the1*m1^2*m2*cos(the1 - the2)^2 - g*m2^3*cos(the1 - the2)*sin(the1)^2*sin(the2) - 2*g*m2^3*sin(the1 - the2)*cos(the2)*sin(the1)^2 + Fx*m1*m2*sin(the1 - the2)^2*cos(the1) + 2*d1l1*d1the1*m*m2^2*sin(the1 - the2)^2 + 4*d1l1*d1the1*m1*m2^2*sin(the1 - the2)^2 + 2*d1l1*d1the1*m1^2*m2*sin(the1 - the2)^2 + d1the2^2*l2*m2^3*cos(the1 - the2)^2*sin(the1 - the2) - d1the2^2*l2*m*m2^2*sin(the1 - the2) - 2*d1the2^2*l2*m1*m2^2*sin(the1 - the2) - d1the2^2*l2*m1^2*m2*sin(the1 - the2) + g*m*m2^2*cos(the1 - the2)*sin(the2) + 2*g*m1*m2^2*cos(the1 - the2)*sin(the2) + g*m1^2*m2*cos(the1 - the2)*sin(the2) - 2*g*m*m1*m2*sin(the1) + g*m*m1*m2*cos(the1 - the2)*sin(the2) - 4*d1l1*d1the1*m1*m2^2*cos(the1 - the2)^2*sin(the1)^2 - 4*d1l1*d1the1*m1*m2^2*sin(the1 - the2)^2*cos(the1)^2 - 2*d1l1*d1the1*m1^2*m2*cos(the1 - the2)^2*sin(the1)^2 - 2*d1l1*d1the1*m1^2*m2*sin(the1 - the2)^2*cos(the1)^2 + d1the2^2*l2*m1*m2^2*sin(the1 - the2)*cos(the2)^2 + d1the2^2*l2*m2^3*cos(the1 - the2)*cos(the1)*sin(the1) + d1the2^2*l2*m2^3*cos(the1 - the2)*cos(the2)*sin(the2) - 2*g*m1*m2^2*sin(the1 - the2)*cos(the1)^2*cos(the2) - g*m1^2*m2*sin(the1 - the2)*cos(the1)^2*cos(the2) + 2*d1the2^2*l2*m1*m2^2*sin(the1 - the2)*sin(the1)^2 + d1the2^2*l2*m1^2*m2*sin(the1 - the2)*sin(the1)^2 - g*m2^3*cos(the1 - the2)*cos(the1)*cos(the2)*sin(the1) - 2*g*m1*m2^2*cos(the1 - the2)*sin(the1)^2*sin(the2) - 4*g*m1*m2^2*sin(the1 - the2)*cos(the2)*sin(the1)^2 - g*m1^2*m2*cos(the1 - the2)*sin(the1)^2*sin(the2) - 2*g*m1^2*m2*sin(the1 - the2)*cos(the2)*sin(the1)^2 - Fl*m1*m2*cos(the1 - the2)*cos(the2)*sin(the1) - Fl*m1*m2*sin(the1 - the2)*cos(the1)*cos(the2) + d1the2^2*l2*m*m2^2*cos(the1 - the2)^2*sin(the1 - the2) + d1the2^2*l2*m1*m2^2*cos(the1 - the2)^2*sin(the1 - the2) + g*m2^3*sin(the1 - the2)*cos(the1)*sin(the1)*sin(the2) + g*m*m1*m2*sin(the1 - the2)^2*sin(the1) - d1the2^2*l2*m2^3*cos(the1 - the2)^2*cos(the2)*sin(the1) - 2*d1the2^2*l2*m1*m2^2*cos(the1)*sin(the2) - d1the2^2*l2*m1^2*m2*cos(the1)*sin(the2) - Fx*m1*m2*cos(the1 - the2)*sin(the1 - the2)*sin(the1) + d1the2^2*l2*m2^3*sin(the1 - the2)^2*cos(the1)*sin(the2) - 2*d1the2^2*l2*m2^3*sin(the1 - the2)^2*cos(the2)*sin(the1) - 2*g*m1*m2^2*cos(the1)*cos(the2)*sin(the2) - g*m1^2*m2*cos(the1)*cos(the2)*sin(the2) - 4*d1l1*d1the1*m2^3*cos(the1 - the2)*cos(the1)*cos(the2) - 4*d1l1*d1the1*m2^3*sin(the1 - the2)*cos(the2)*sin(the1) + 2*d1l1*d1the1*m*m1*m2*cos(the1 - the2)^2 + 2*d1l1*d1the1*m*m1*m2*sin(the1 - the2)^2 - d1the2^2*l2*m*m1*m2*sin(the1 - the2) + g*m*m2^2*cos(the1 - the2)*sin(the1 - the2)*cos(the1) + 2*g*m1*m2^2*cos(the1 - the2)*sin(the1 - the2)*cos(the1) + g*m1^2*m2*cos(the1 - the2)*sin(the1 - the2)*cos(the1) + d1the2^2*l2*m1*m2^2*sin(the1 - the2)^2*cos(the1)*sin(the2) - 2*d1the2^2*l2*m1*m2^2*sin(the1 - the2)^2*cos(the2)*sin(the1) + g*m*m1*m2*cos(the1 - the2)*sin(the1 - the2)*cos(the1) - 8*d1l1*d1the1*m1*m2^2*cos(the1 - the2)*cos(the1)*cos(the2) - 4*d1l1*d1the1*m1^2*m2*cos(the1 - the2)*cos(the1)*cos(the2) - d1the2^2*l2*m2^3*cos(the1 - the2)*sin(the1 - the2)*cos(the1)*cos(the2) - 8*d1l1*d1the1*m1*m2^2*sin(the1 - the2)*cos(the2)*sin(the1) - 4*d1l1*d1the1*m1^2*m2*sin(the1 - the2)*cos(the2)*sin(the1) - d1the2^2*l2*m2^3*cos(the1 - the2)*sin(the1 - the2)*sin(the1)*sin(the2) + 2*d1the2^2*l2*m1*m2^2*cos(the1 - the2)*cos(the1)*sin(the1) + d1the2^2*l2*m1^2*m2*cos(the1 - the2)*cos(the1)*sin(the1) + d1the2^2*l2*m1*m2^2*cos(the1 - the2)*cos(the2)*sin(the2) - 2*g*m1*m2^2*cos(the1 - the2)*cos(the1)*cos(the2)*sin(the1) - g*m1^2*m2*cos(the1 - the2)*cos(the1)*cos(the2)*sin(the1) + 2*g*m1*m2^2*sin(the1 - the2)*cos(the1)*sin(the1)*sin(the2) + g*m1^2*m2*sin(the1 - the2)*cos(the1)*sin(the1)*sin(the2) + 4*d1l1*d1the1*m2^3*cos(the1 - the2)*sin(the1 - the2)*cos(the1)*sin(the1) - d1the2^2*l2*m1*m2^2*cos(the1 - the2)^2*cos(the2)*sin(the1) + 8*d1l1*d1the1*m1*m2^2*cos(the1 - the2)*sin(the1 - the2)*cos(the1)*sin(the1) + 4*d1l1*d1the1*m1^2*m2*cos(the1 - the2)*sin(the1 - the2)*cos(the1)*sin(the1) - d1the2^2*l2*m1*m2^2*cos(the1 - the2)*sin(the1 - the2)*cos(the1)*cos(the2) - d1the2^2*l2*m1*m2^2*cos(the1 - the2)*sin(the1 - the2)*sin(the1)*sin(the2))/(l1*(m1 + m2)*(m1^2*cos(the1)^2 - m*m2 - 2*m1*m2 - m*m1 + m2^2*cos(the1)^2 + m2^2*cos(the2)^2 + m1^2*sin(the1)^2 + m2^2*sin(the1)^2 + m2^2*cos(the1 - the2)^2 + m2^2*sin(the1 - the2)^2 - m1^2 - m2^2 + 2*m1*m2*cos(the1)^2 + m1*m2*cos(the2)^2 + 2*m1*m2*sin(the1)^2 + m*m2*cos(the1 - the2)^2 + m1*m2*cos(the1 - the2)^2 + m*m2*sin(the1 - the2)^2 + m1*m2*sin(the1 - the2)^2 - m2^2*cos(the1 - the2)^2*sin(the1)^2 - m2^2*sin(the1 - the2)^2*cos(the1)^2 - 2*m2^2*sin(the1 - the2)*cos(the2)*sin(the1) - 2*m2^2*cos(the1 - the2)*cos(the1)*cos(the2) - m1*m2*cos(the1 - the2)^2*sin(the1)^2 - m1*m2*sin(the1 - the2)^2*cos(the1)^2 + 2*m2^2*cos(the1 - the2)*sin(the1 - the2)*cos(the1)*sin(the1) - 2*m1*m2*sin(the1 - the2)*cos(the2)*sin(the1) - 2*m1*m2*cos(the1 - the2)*cos(the1)*cos(the2) + 2*m1*m2*cos(the1 - the2)*sin(the1 - the2)*cos(the1)*sin(the1)));

 %dx6 = -(2*d1l1*d1the1*m1^3*cos(the1)^2 - Fx*m2^2*cos(the1) - 2*d1l1*d1the1*m1^3 - 2*d1l1*d1the1*m2^3 - Fx*m1^2*cos(the1) + 2*d1l1*d1the1*m2^3*cos(the1)^2 + 2*d1l1*d1the1*m2^3*cos(the2)^2 + Fl*m1^2*cos(the1)*sin(the1) + Fl*m2^2*cos(the1)*sin(the1) + 2*d1l1*d1the1*m1^3*sin(the1)^2 + 2*d1l1*d1the1*m2^3*sin(the1)^2 - g*m1^3*cos(the1)*sin(the1) - g*m2^3*cos(the1)*sin(the1) + Fx*m2^2*cos(the1 - the2)*cos(the2) - 2*Fx*m1*m2*cos(the1) + 2*d1l1*d1the1*m2^4*cos(the1 - the2)^2 - 2*d1l1*d1the1*m*m1^2 - 2*d1l1*d1the1*m*m2^2 - 6*d1l1*d1the1*m1*m2^2 - 6*d1l1*d1the1*m1^2*m2 + 2*d1l1*d1the1*m2^3*sin(the1 - the2)^2 - d1the2^2*l2*m2^3*sin(the1 - the2) + g*m2^3*cos(the1 - the2)*sin(the2) + Fl*m2^2*cos(the1 - the2)*sin(the1 - the2) + g*m1^3*cos(the1)^2*sin(the1) + g*m2^3*cos(the1)^2*sin(the1) - g*m2^3*cos(the1 - the2)*sin(the1 - the2) + Fx*m2^2*sin(the1 - the2)^2*cos(the1) + d1the2^2*l2*m2^3*sin(the1 - the2)^3 - d1the2^2*l2*m2^3*cos(the1)*sin(the2) + 3*g*m1*m2^2*cos(the1)^2*sin(the1) + 3*g*m1^2*m2*cos(the1)^2*sin(the1) - g*m*m2^2*cos(the1 - the2)*sin(the1 - the2) - 2*g*m1*m2^2*cos(the1 - the2)*sin(the1 - the2) - g*m1^2*m2*cos(the1 - the2)*sin(the1 - the2) - g*m2^3*cos(the1)*cos(the2)*sin(the2) + 2*d1l1*d1the1*m1^2*m2^2*cos(the1 - the2)^2 - Fl*m2^2*cos(the1 - the2)*cos(the2)*sin(the1) - Fl*m2^2*sin(the1 - the2)*cos(the1)*cos(the2) + 2*Fl*m1*m2*cos(the1)*sin(the1) + d1the2^2*l2*m*m2^2*sin(the1 - the2)^3 + d1the2^2*l2*m1*m2^2*sin(the1 - the2)^3 + g*m2^3*cos(the1 - the2)*cos(the2)*sin(the1) + g*m2^3*sin(the1 - the2)*cos(the1)*cos(the2) + Fx*m1*m2*cos(the1 - the2)*cos(the2) - 4*d1l1*d1the1*m*m1*m2 - Fx*m2^2*cos(the1 - the2)*sin(the1 - the2)*sin(the1) + g*m2^3*cos(the1 - the2)*sin(the1 - the2)*cos(the1) + 6*d1l1*d1the1*m1*m2^2*cos(the1)^2 + 6*d1l1*d1the1*m1^2*m2*cos(the1)^2 + 4*d1l1*d1the1*m1*m2^2*cos(the2)^2 + 2*d1l1*d1the1*m1^2*m2*cos(the2)^2 - 2*d1l1*d1the1*m2^3*sin(the1 - the2)^2*cos(the1)^2 - 2*d1l1*d1the1*m2^4*cos(the1 - the2)^2*sin(the1)^2 + Fl*m*m2*cos(the1 - the2)*sin(the1 - the2) + Fl*m1*m2*cos(the1 - the2)*sin(the1 - the2) + 6*d1l1*d1the1*m1*m2^2*sin(the1)^2 + 6*d1l1*d1the1*m1^2*m2*sin(the1)^2 + d1the2^2*l2*m2^3*sin(the1 - the2)*cos(the2)^2 - g*m2^3*sin(the1 - the2)*cos(the1)^2*cos(the2) + d1the2^2*l2*m2^3*sin(the1 - the2)*sin(the1)^2 - 3*g*m1*m2^2*cos(the1)*sin(the1) - 3*g*m1^2*m2*cos(the1)*sin(the1) + 2*d1l1*d1the1*m*m2^3*cos(the1 - the2)^2 + 4*d1l1*d1the1*m1*m2^3*cos(the1 - the2)^2 - g*m2^3*cos(the1 - the2)*sin(the1)^2*sin(the2) + Fx*m1*m2*sin(the1 - the2)^2*cos(the1) + 2*d1l1*d1the1*m*m2^2*sin(the1 - the2)^2 + 4*d1l1*d1the1*m1*m2^2*sin(the1 - the2)^2 + 2*d1l1*d1the1*m1^2*m2*sin(the1 - the2)^2 - d1the2^2*l2*m2^3*cos(the1 - the2)^2*sin(the1 - the2) - d1the2^2*l2*m*m2^2*sin(the1 - the2) - 2*d1the2^2*l2*m1*m2^2*sin(the1 - the2) - d1the2^2*l2*m1^2*m2*sin(the1 - the2) + g*m*m2^2*cos(the1 - the2)*sin(the2) + 2*g*m1*m2^2*cos(the1 - the2)*sin(the2) + g*m1^2*m2*cos(the1 - the2)*sin(the2) + g*m*m1*m2*cos(the1 - the2)*sin(the2) - 4*d1l1*d1the1*m1*m2^2*sin(the1 - the2)^2*cos(the1)^2 - 2*d1l1*d1the1*m1^2*m2*sin(the1 - the2)^2*cos(the1)^2 - 4*d1l1*d1the1*m1*m2^3*cos(the1 - the2)^2*sin(the1)^2 + d1the2^2*l2*m1*m2^2*sin(the1 - the2)*cos(the2)^2 - d1the2^2*l2*m2^3*cos(the1 - the2)*cos(the1)*sin(the1) + d1the2^2*l2*m2^3*cos(the1 - the2)*cos(the2)*sin(the2) - 2*g*m1*m2^2*sin(the1 - the2)*cos(the1)^2*cos(the2) - g*m1^2*m2*sin(the1 - the2)*cos(the1)^2*cos(the2) + 2*d1the2^2*l2*m1*m2^2*sin(the1 - the2)*sin(the1)^2 + d1the2^2*l2*m1^2*m2*sin(the1 - the2)*sin(the1)^2 - g*m*m1*m2*cos(the1 - the2)*sin(the1 - the2) - g*m2^3*cos(the1 - the2)*cos(the1)*cos(the2)*sin(the1) + 2*d1l1*d1the1*m*m1*m2^2*cos(the1 - the2)^2 - 2*g*m1*m2^2*cos(the1 - the2)*sin(the1)^2*sin(the2) - g*m1^2*m2*cos(the1 - the2)*sin(the1)^2*sin(the2) - Fl*m1*m2*cos(the1 - the2)*cos(the2)*sin(the1) - Fl*m1*m2*sin(the1 - the2)*cos(the1)*cos(the2) - d1the2^2*l2*m*m2^2*cos(the1 - the2)^2*sin(the1 - the2) - d1the2^2*l2*m1*m2^2*cos(the1 - the2)^2*sin(the1 - the2) + g*m2^3*sin(the1 - the2)*cos(the1)*sin(the1)*sin(the2) - 2*d1l1*d1the1*m1^2*m2^2*cos(the1 - the2)^2*sin(the1)^2 + d1the2^2*l2*m2^3*cos(the1 - the2)^2*cos(the2)*sin(the1) - 2*d1the2^2*l2*m1*m2^2*cos(the1)*sin(the2) - d1the2^2*l2*m1^2*m2*cos(the1)*sin(the2) - Fx*m1*m2*cos(the1 - the2)*sin(the1 - the2)*sin(the1) + d1the2^2*l2*m2^3*sin(the1 - the2)^2*cos(the1)*sin(the2) - 2*d1the2^2*l2*m2^3*sin(the1 - the2)^2*cos(the2)*sin(the1) - 2*g*m1*m2^2*cos(the1)*cos(the2)*sin(the2) - g*m1^2*m2*cos(the1)*cos(the2)*sin(the2) - 2*d1l1*d1the1*m2^3*cos(the1 - the2)*cos(the1)*cos(the2) - 2*d1l1*d1the1*m2^4*cos(the1 - the2)*cos(the1)*cos(the2) + 2*g*m1*m2^2*cos(the1 - the2)*cos(the2)*sin(the1) + 2*g*m1*m2^2*sin(the1 - the2)*cos(the1)*cos(the2) + g*m1^2*m2*cos(the1 - the2)*cos(the2)*sin(the1) + g*m1^2*m2*sin(the1 - the2)*cos(the1)*cos(the2) - 4*d1l1*d1the1*m2^3*sin(the1 - the2)*cos(the2)*sin(the1) + 2*d1l1*d1the1*m*m1*m2*sin(the1 - the2)^2 - d1the2^2*l2*m*m1*m2*sin(the1 - the2) + g*m*m2^2*cos(the1 - the2)*sin(the1 - the2)*cos(the1) + 2*g*m1*m2^2*cos(the1 - the2)*sin(the1 - the2)*cos(the1) + g*m1^2*m2*cos(the1 - the2)*sin(the1 - the2)*cos(the1) + d1the2^2*l2*m1*m2^2*sin(the1 - the2)^2*cos(the1)*sin(the2) - 2*d1the2^2*l2*m1*m2^2*sin(the1 - the2)^2*cos(the2)*sin(the1) + g*m*m1*m2*cos(the1 - the2)*sin(the1 - the2)*cos(the1) - 4*d1l1*d1the1*m1*m2^2*cos(the1 - the2)*cos(the1)*cos(the2) - 2*d1l1*d1the1*m1^2*m2*cos(the1 - the2)*cos(the1)*cos(the2) - 4*d1l1*d1the1*m1*m2^3*cos(the1 - the2)*cos(the1)*cos(the2) + d1the2^2*l2*m2^3*cos(the1 - the2)*sin(the1 - the2)*cos(the1)*cos(the2) - 8*d1l1*d1the1*m1*m2^2*sin(the1 - the2)*cos(the2)*sin(the1) - 4*d1l1*d1the1*m1^2*m2*sin(the1 - the2)*cos(the2)*sin(the1) - d1the2^2*l2*m2^3*cos(the1 - the2)*sin(the1 - the2)*sin(the1)*sin(the2) - 2*d1l1*d1the1*m1^2*m2^2*cos(the1 - the2)*cos(the1)*cos(the2) - 2*d1the2^2*l2*m1*m2^2*cos(the1 - the2)*cos(the1)*sin(the1) - d1the2^2*l2*m1^2*m2*cos(the1 - the2)*cos(the1)*sin(the1) + d1the2^2*l2*m1*m2^2*cos(the1 - the2)*cos(the2)*sin(the2) - 2*g*m1*m2^2*cos(the1 - the2)*cos(the1)*cos(the2)*sin(the1) - g*m1^2*m2*cos(the1 - the2)*cos(the1)*cos(the2)*sin(the1) + 2*g*m1*m2^2*sin(the1 - the2)*cos(the1)*sin(the1)*sin(the2) + g*m1^2*m2*sin(the1 - the2)*cos(the1)*sin(the1)*sin(the2) + 2*d1l1*d1the1*m2^3*cos(the1 - the2)*sin(the1 - the2)*cos(the1)*sin(the1) + 2*d1l1*d1the1*m2^4*cos(the1 - the2)*sin(the1 - the2)*cos(the1)*sin(the1) + d1the2^2*l2*m1*m2^2*cos(the1 - the2)^2*cos(the2)*sin(the1) + 4*d1l1*d1the1*m1*m2^2*cos(the1 - the2)*sin(the1 - the2)*cos(the1)*sin(the1) + 2*d1l1*d1the1*m1^2*m2*cos(the1 - the2)*sin(the1 - the2)*cos(the1)*sin(the1) + 4*d1l1*d1the1*m1*m2^3*cos(the1 - the2)*sin(the1 - the2)*cos(the1)*sin(the1) + d1the2^2*l2*m1*m2^2*cos(the1 - the2)*sin(the1 - the2)*cos(the1)*cos(the2) + 2*d1l1*d1the1*m1^2*m2^2*cos(the1 - the2)*sin(the1 - the2)*cos(the1)*sin(the1) - d1the2^2*l2*m1*m2^2*cos(the1 - the2)*sin(the1 - the2)*sin(the1)*sin(the2))/(l1*(m1 + m2)*(m1^2*cos(the1)^2 - m*m2 - 2*m1*m2 - m*m1 + m2^2*cos(the1)^2 + m2^2*cos(the2)^2 + m1^2*sin(the1)^2 + m2^2*sin(the1)^2 + m2^2*cos(the1 - the2)^2 + m2^2*sin(the1 - the2)^2 - m1^2 - m2^2 + 2*m1*m2*cos(the1)^2 + m1*m2*cos(the2)^2 + 2*m1*m2*sin(the1)^2 + m*m2*cos(the1 - the2)^2 + m1*m2*cos(the1 - the2)^2 + m*m2*sin(the1 - the2)^2 + m1*m2*sin(the1 - the2)^2 - m2^2*cos(the1 - the2)^2*sin(the1)^2 - m2^2*sin(the1 - the2)^2*cos(the1)^2 - 2*m2^2*sin(the1 - the2)*cos(the2)*sin(the1) - 2*m2^2*cos(the1 - the2)*cos(the1)*cos(the2) - m1*m2*cos(the1 - the2)^2*sin(the1)^2 - m1*m2*sin(the1 - the2)^2*cos(the1)^2 + 2*m2^2*cos(the1 - the2)*sin(the1 - the2)*cos(the1)*sin(the1) - 2*m1*m2*sin(the1 - the2)*cos(the2)*sin(the1) - 2*m1*m2*cos(the1 - the2)*cos(the1)*cos(the2) + 2*m1*m2*cos(the1 - the2)*sin(the1 - the2)*cos(the1)*sin(the1)));

 dx7=d1the2;

 dx8 = -(Fx*m1*sin(the1 - the2)*sin(the1) - Fl*m1*sin(the1 - the2) - Fl*m2*sin(the1 - the2) - g*m1^2*sin(the2) - g*m2^2*sin(the2) - Fx*m1*cos(the2) - Fx*m2*cos(the2) - Fl*m*sin(the1 - the2) + Fx*m2*sin(the1 - the2)*sin(the1) + Fl*m1*sin(the1 - the2)*cos(the1)^2 + Fl*m2*sin(the1 - the2)*cos(the1)^2 + g*m1^2*cos(the1 - the2)*sin(the1) - g*m1^2*sin(the1 - the2)*cos(the1) + g*m2^2*cos(the1 - the2)*sin(the1) - g*m2^2*sin(the1 - the2)*cos(the1) - g*m*m1*sin(the2) - g*m*m2*sin(the2) - 2*g*m1*m2*sin(the2) + g*m1^2*cos(the1)^2*sin(the2) + g*m2^2*cos(the1)^2*sin(the2) + g*m1^2*sin(the1)^2*sin(the2) + g*m2^2*sin(the1)^2*sin(the2) + Fl*m1*cos(the2)*sin(the1) + Fl*m2*cos(the2)*sin(the1) - g*m1^2*cos(the1 - the2)*sin(the1)^3 + g*m1^2*sin(the1 - the2)*cos(the1)^3 - g*m2^2*cos(the1 - the2)*sin(the1)^3 + g*m2^2*sin(the1 - the2)*cos(the1)^3 + Fx*m1*cos(the1 - the2)*cos(the1) + Fx*m2*cos(the1 - the2)*cos(the1) - d1the2^2*l2*m2^2*cos(the2)*sin(the2) + g*m*m1*cos(the1 - the2)*sin(the1) - g*m*m1*sin(the1 - the2)*cos(the1) + g*m*m2*cos(the1 - the2)*sin(the1) - g*m*m2*sin(the1 - the2)*cos(the1) + 2*g*m1*m2*cos(the1 - the2)*sin(the1) - 2*g*m1*m2*sin(the1 - the2)*cos(the1) - g*m1^2*cos(the1 - the2)*cos(the1)^2*sin(the1) - g*m2^2*cos(the1 - the2)*cos(the1)^2*sin(the1) + 2*g*m1*m2*cos(the1)^2*sin(the2) + g*m1^2*sin(the1 - the2)*cos(the1)*sin(the1)^2 + g*m2^2*sin(the1 - the2)*cos(the1)*sin(the1)^2 + 2*g*m1*m2*sin(the1)^2*sin(the2) - Fl*m1*cos(the1 - the2)*cos(the1)*sin(the1) - Fl*m2*cos(the1 - the2)*cos(the1)*sin(the1) - 2*g*m1*m2*cos(the1 - the2)*sin(the1)^3 + 2*g*m1*m2*sin(the1 - the2)*cos(the1)^3 + d1the2^2*l2*m2^2*cos(the1 - the2)*cos(the1)*sin(the2) + d1the2^2*l2*m2^2*cos(the1 - the2)*cos(the2)*sin(the1) - d1the2^2*l2*m2^2*sin(the1 - the2)*cos(the1)*cos(the2) - d1the2^2*l2*m1*m2*cos(the2)*sin(the2) + d1the2^2*l2*m2^2*sin(the1 - the2)*sin(the1)*sin(the2) - d1the2^2*l2*m2^2*cos(the1 - the2)^2*cos(the1)*sin(the1) + d1the2^2*l2*m2^2*sin(the1 - the2)^2*cos(the1)*sin(the1) + d1the2^2*l2*m2^2*cos(the1 - the2)*sin(the1 - the2)*cos(the1)^2 - d1the2^2*l2*m2^2*cos(the1 - the2)*sin(the1 - the2)*sin(the1)^2 - 2*g*m1*m2*cos(the1 - the2)*cos(the1)^2*sin(the1) + 2*g*m1*m2*sin(the1 - the2)*cos(the1)*sin(the1)^2 + d1the2^2*l2*m1*m2*cos(the1 - the2)*cos(the1)*sin(the2) + d1the2^2*l2*m1*m2*cos(the1 - the2)*cos(the2)*sin(the1) - d1the2^2*l2*m1*m2*sin(the1 - the2)*cos(the1)*cos(the2) + d1the2^2*l2*m1*m2*sin(the1 - the2)*sin(the1)*sin(the2) - d1the2^2*l2*m1*m2*cos(the1 - the2)^2*cos(the1)*sin(the1) + d1the2^2*l2*m1*m2*sin(the1 - the2)^2*cos(the1)*sin(the1) + d1the2^2*l2*m1*m2*cos(the1 - the2)*sin(the1 - the2)*cos(the1)^2 - d1the2^2*l2*m1*m2*cos(the1 - the2)*sin(the1 - the2)*sin(the1)^2)/(l2*(m1^2*cos(the1)^2 - m*m2 - 2*m1*m2 - m*m1 + m2^2*cos(the1)^2 + m2^2*cos(the2)^2 + m1^2*sin(the1)^2 + m2^2*sin(the1)^2 + m2^2*cos(the1 - the2)^2 + m2^2*sin(the1 - the2)^2 - m1^2 - m2^2 + 2*m1*m2*cos(the1)^2 + m1*m2*cos(the2)^2 + 2*m1*m2*sin(the1)^2 + m*m2*cos(the1 - the2)^2 + m1*m2*cos(the1 - the2)^2 + m*m2*sin(the1 - the2)^2 + m1*m2*sin(the1 - the2)^2 - m2^2*cos(the1 - the2)^2*sin(the1)^2 - m2^2*sin(the1 - the2)^2*cos(the1)^2 - 2*m2^2*sin(the1 - the2)*cos(the2)*sin(the1) - 2*m2^2*cos(the1 - the2)*cos(the1)*cos(the2) - m1*m2*cos(the1 - the2)^2*sin(the1)^2 - m1*m2*sin(the1 - the2)^2*cos(the1)^2 + 2*m2^2*cos(the1 - the2)*sin(the1 - the2)*cos(the1)*sin(the1) - 2*m1*m2*sin(the1 - the2)*cos(the2)*sin(the1) - 2*m1*m2*cos(the1 - the2)*cos(the1)*cos(the2) + 2*m1*m2*cos(the1 - the2)*sin(the1 - the2)*cos(the1)*sin(the1)));

 %dx8 = -(g*m1^2*sin(the1 - the2) - Fl*m1*sin(the1 - the2) - Fl*m2*sin(the1 - the2) - g*m1^2*sin(the2) - g*m2^2*sin(the2) - Fl*m*sin(the1 - the2) + g*m2^2*sin(the1 - the2) - Fx*m1*cos(the2) - Fx*m2*cos(the2) + Fx*m1*sin(the1 - the2)*sin(the1) + Fx*m2*sin(the1 - the2)*sin(the1) - g*m1^2*cos(the2)*sin(the1) - g*m2^2*cos(the2)*sin(the1) + Fl*m1*sin(the1 - the2)*cos(the1)^2 + Fl*m2*sin(the1 - the2)*cos(the1)^2 - g*m1^2*sin(the1 - the2)*cos(the1) - g*m2^2*sin(the1 - the2)*cos(the1) - g*m*m1*sin(the2) - g*m*m2*sin(the2) - 2*g*m1*m2*sin(the2) + g*m1^2*cos(the1)^2*sin(the2) + g*m2^2*cos(the1)^2*sin(the2) + g*m*m1*sin(the1 - the2) + g*m*m2*sin(the1 - the2) + 2*g*m1*m2*sin(the1 - the2) + g*m1^2*sin(the1)^2*sin(the2) + g*m2^2*sin(the1)^2*sin(the2) + Fl*m1*cos(the2)*sin(the1) + Fl*m2*cos(the2)*sin(the1) - g*m1^2*sin(the1 - the2)*cos(the1)^2 + g*m1^2*sin(the1 - the2)*cos(the1)^3 - g*m2^2*sin(the1 - the2)*cos(the1)^2 + g*m2^2*sin(the1 - the2)*cos(the1)^3 + Fx*m1*cos(the1 - the2)*cos(the1) + Fx*m2*cos(the1 - the2)*cos(the1) + 2*d1l1*d1the1*m1^2*cos(the1 - the2) + 2*d1l1*d1the1*m2^2*cos(the1 - the2) - 2*d1l1*d1the1*m2^3*cos(the1 - the2) + 2*d1l1*d1the1*m*m1*cos(the1 - the2) + 2*d1l1*d1the1*m*m2*cos(the1 - the2) + 4*d1l1*d1the1*m1*m2*cos(the1 - the2) - d1the2^2*l2*m2^2*cos(the2)*sin(the2) + g*m1^2*cos(the1)*cos(the2)*sin(the1) + g*m2^2*cos(the1)*cos(the2)*sin(the1) - 2*d1l1*d1the1*m1^2*cos(the1 - the2)*cos(the1)^2 - 2*d1l1*d1the1*m2^2*cos(the1 - the2)*cos(the1)^2 + 2*d1l1*d1the1*m2^3*cos(the1 - the2)*cos(the1)^2 - 2*d1l1*d1the1*m1^2*cos(the1 - the2)*sin(the1)^2 - 2*d1l1*d1the1*m2^2*cos(the1 - the2)*sin(the1)^2 + 2*d1l1*d1the1*m2^3*cos(the1 - the2)*sin(the1)^2 + g*m1^2*cos(the1 - the2)*cos(the1)*sin(the1) + g*m2^2*cos(the1 - the2)*cos(the1)*sin(the1) - 2*g*m1*m2*cos(the2)*sin(the1) - 2*d1l1*d1the1*m*m2^2*cos(the1 - the2) - 4*d1l1*d1the1*m1*m2^2*cos(the1 - the2) - 2*d1l1*d1the1*m1^2*m2*cos(the1 - the2) + 2*d1the2^2*l2*m2^2*cos(the1 - the2)*sin(the1 - the2) - g*m*m1*sin(the1 - the2)*cos(the1) - g*m*m2*sin(the1 - the2)*cos(the1) - 2*g*m1*m2*sin(the1 - the2)*cos(the1) - g*m1^2*cos(the1 - the2)*cos(the1)^2*sin(the1) - g*m2^2*cos(the1 - the2)*cos(the1)^2*sin(the1) + 2*g*m1*m2*cos(the1)^2*sin(the2) + 2*g*m1*m2*sin(the1)^2*sin(the2) - Fl*m1*cos(the1 - the2)*cos(the1)*sin(the1) - Fl*m2*cos(the1 - the2)*cos(the1)*sin(the1) - 2*g*m1*m2*sin(the1 - the2)*cos(the1)^2 + 2*g*m1*m2*sin(the1 - the2)*cos(the1)^3 + d1the2^2*l2*m2^2*cos(the1 - the2)*cos(the1)*sin(the2) - d1the2^2*l2*m2^2*cos(the1 - the2)*cos(the2)*sin(the1) - d1the2^2*l2*m2^2*sin(the1 - the2)*cos(the1)*cos(the2) - d1the2^2*l2*m1*m2*cos(the2)*sin(the2) + 2*g*m1*m2*cos(the1)*cos(the2)*sin(the1) - 4*d1l1*d1the1*m1*m2*cos(the1 - the2)*cos(the1)^2 + d1the2^2*l2*m2^2*sin(the1 - the2)*sin(the1)*sin(the2) - 4*d1l1*d1the1*m1*m2*cos(the1 - the2)*sin(the1)^2 + 2*g*m1*m2*cos(the1 - the2)*cos(the1)*sin(the1) - 2*d1l1*d1the1*m*m1*m2*cos(the1 - the2) + d1the2^2*l2*m2^2*cos(the1 - the2)^2*cos(the1)*sin(the1) + 2*d1the2^2*l2*m*m2*cos(the1 - the2)*sin(the1 - the2) + 2*d1the2^2*l2*m1*m2*cos(the1 - the2)*sin(the1 - the2) + d1the2^2*l2*m2^2*sin(the1 - the2)^2*cos(the1)*sin(the1) + 4*d1l1*d1the1*m1*m2^2*cos(the1 - the2)*cos(the1)^2 + 2*d1l1*d1the1*m1^2*m2*cos(the1 - the2)*cos(the1)^2 + 4*d1l1*d1the1*m1*m2^2*cos(the1 - the2)*sin(the1)^2 + 2*d1l1*d1the1*m1^2*m2*cos(the1 - the2)*sin(the1)^2 - d1the2^2*l2*m2^2*cos(the1 - the2)*sin(the1 - the2)*cos(the1)^2 - d1the2^2*l2*m2^2*cos(the1 - the2)*sin(the1 - the2)*sin(the1)^2 - 2*g*m1*m2*cos(the1 - the2)*cos(the1)^2*sin(the1) + d1the2^2*l2*m1*m2*cos(the1 - the2)*cos(the1)*sin(the2) - d1the2^2*l2*m1*m2*cos(the1 - the2)*cos(the2)*sin(the1) - d1the2^2*l2*m1*m2*sin(the1 - the2)*cos(the1)*cos(the2) + d1the2^2*l2*m1*m2*sin(the1 - the2)*sin(the1)*sin(the2) + d1the2^2*l2*m1*m2*cos(the1 - the2)^2*cos(the1)*sin(the1) + d1the2^2*l2*m1*m2*sin(the1 - the2)^2*cos(the1)*sin(the1) - d1the2^2*l2*m1*m2*cos(the1 - the2)*sin(the1 - the2)*cos(the1)^2 - d1the2^2*l2*m1*m2*cos(the1 - the2)*sin(the1 - the2)*sin(the1)^2)/(l2*(m1^2*cos(the1)^2 - m*m2 - 2*m1*m2 - m*m1 + m2^2*cos(the1)^2 + m2^2*cos(the2)^2 + m1^2*sin(the1)^2 + m2^2*sin(the1)^2 + m2^2*cos(the1 - the2)^2 + m2^2*sin(the1 - the2)^2 - m1^2 - m2^2 + 2*m1*m2*cos(the1)^2 + m1*m2*cos(the2)^2 + 2*m1*m2*sin(the1)^2 + m*m2*cos(the1 - the2)^2 + m1*m2*cos(the1 - the2)^2 + m*m2*sin(the1 - the2)^2 + m1*m2*sin(the1 - the2)^2 - m2^2*cos(the1 - the2)^2*sin(the1)^2 - m2^2*sin(the1 - the2)^2*cos(the1)^2 - 2*m2^2*sin(the1 - the2)*cos(the2)*sin(the1) - 2*m2^2*cos(the1 - the2)*cos(the1)*cos(the2) - m1*m2*cos(the1 - the2)^2*sin(the1)^2 - m1*m2*sin(the1 - the2)^2*cos(the1)^2 + 2*m2^2*cos(the1 - the2)*sin(the1 - the2)*cos(the1)*sin(the1) - 2*m1*m2*sin(the1 - the2)*cos(the2)*sin(the1) - 2*m1*m2*cos(the1 - the2)*cos(the1)*cos(the2) + 2*m1*m2*cos(the1 - the2)*sin(the1 - the2)*cos(the1)*sin(the1)));
